simulink model "EcoSIM3_P2_C2"  (R2014b)
settings: Solver=ode1  SolverMode=SingleTasking  StartTime=0.0  StopTime=inf  FixedStep=0.01  RelTol=1e-3
PostLoadFcn:
  | %, if any(exist('dsrtsu_mdlpostloadfcn', 'file') == [2, 3, 6]), try dsrtsu_mdlpostloadfcn('Execute', bdroot); catch fprintf('Error in PostLoadFcn (dsrtsu_mdlpostloadfcn) for model "%s":\n %s\n', bdroot, lasterr); end, end,
InitFcn:
  | tic
  | %Startup_EcoSIM
values from neighbouring files (symbols this model uses):
  EngPwr = [0 5	10	15	20	25	30	35	40	45	50	55	60	65	70	75	80	85	90	95	100	105	110	115]    [Series_Maps.m]
  EngSpd = [0 477.4645 954.929 1909.858 2864.787 3819.716 4774.645 5729.574 6684.503]    [Series_Maps.m]
  EngTrq = [0	0	0	0	0	0	0	0	0	0	0	0	0	0	0	0	0	0	0	0	0	0	0	0 ... (first row only)    [Series_Maps.m]
  Power = [0 5 10 15 20 25 30]    [Series_Maps.m]
  Torque = [-50,-40,-30,-25,-20,-15,-10,-8,-6,-4,-2,0]    [Series_Maps.m]
undefined symbols (not defined in the file or in its folder): canChannel, Controls, DriveCycles, Driver, EM_EFF_MAP, EM_PwrLoss_MAP, Glbl, Plants, Veh_Dynamics
libraries: canmsglib x100, canlib x87, fl_lib x78, simulink x59, nesl_utility x40, sdl_lib x17, dspsigops x5, dspswit3 x3, dspstat3 x2, commnoisgen2 x1, dspfdesign x1
(part 5 of 15)

== system EcoSIM3_P2_C2/Powertrain/Electrical Storage System/Soft ECU/Outputs ==
  note: Select the Sensor signals
  From Algorithm : Inport
  Bus Creator2 : BusCreator  Inputs=6
  Bus Creator3 : BusCreator  Inputs=2
  Bus Selector : BusSelector  OutputSignals=AccPwrMdlHiVltInpCrnt,bcm_mainc_stat,Batt_SOC_percent,SoftECU_Out,Batt_Voltage_V,Batt_Current_A,bcm_cell_tmax,bcm_cell_tmin
  Actuator_Cmds : Outport
  To ECUs : Outport  Port=2
  wires:
  Bus Selector/4 -> Bus Creator2/2  "<SoftECU_Out>"
  Bus Selector/3 -> Bus Creator2/1  "<Batt_SOC_percent>"
  Bus Selector/2 -> Bus Creator3/2  "<bcm_mainc_stat>"
  Bus Selector/1 -> Bus Creator3/1  "<AccPwrMdlHiVltInpCrnt>"
  From Algorithm/1 -> Bus Selector/1
  Bus Creator2/1 -> To ECUs/1  "ESS_CAN_Out"
  Bus Creator3/1 -> Actuator_Cmds/1  "ESS_Actuator_Cmds"
  Bus Selector/5 -> Bus Creator2/3  "<Batt_Voltage_V>"
  Bus Selector/6 -> Bus Creator2/4  "<Batt_Current_A>"
  Bus Selector/7 -> Bus Creator2/5  "<bcm_cell_tmax>"
  Bus Selector/8 -> Bus Creator2/6  "<bcm_cell_tmin>"

== system EcoSIM3_P2_C2/Powertrain/Engine/ Component Model/Actuators ==
  note: Actuator Model or a Signal Pass-through, Remove the bus if you are passing through all the signals
  ActuatorInputs : Inport
  Actuator Outputs : Outport
  wires:
  ActuatorInputs/1 -> Actuator Outputs/1

== system EcoSIM3_P2_C2/Powertrain/Engine/ Component Model/Plant ==
  note: Component Level Performance Maps
  note: Three kinds of Outputs:
      | 1.To_sensors: Signals that can actually be sensed through Sensors go to sensor models
      | 2. To_plants: Signals that are not actually sensed by sensors but are utilized by the rest of the plant and actually happen physically
      | Component_Logging: Logs both the signal kinds before going through sensor
  From_Actuators : Inport
  Sensors_Feedback : Inport  Port=2
  Bus Selector : BusSelector  OutputSignals=ICE_Torque_Cmd_Nm
  Bus Selector1 : BusSelector  OutputSignals=ICE_Speed_rad_per_s
  Compare To Constant : simulink/Logic and Bit Operations/Compare To Constant  relop=>=  const=0  OutDataTypeStr=boolean
  Generic Engine : sdl_lib/Engines/Generic Engine  Commented=on  model_parameterization=1  engine_type=1  P_max=max(Plants.ICE.Mdl.Plant.Max_Trq.Trq.*Plants.ICE.Mdl.Plant.Max_Trq.w) W  w_P_max=6000 rpm  w_max="max(Plants.ICE.Mdl.Plant.Max_Trq.RPM)  rpm"  w_min="min(Plants.ICE.Mdl.Plant.Max_Trq.RPM)  rpm"  w_tab=[ 500 1000 2e+3 3e+3 4e+3 5e+3 6e+3 7e+3 ] rpm  trq_tab=[ 380 380 380 380 350 280 200 80 ] N*m  pwr_tab=[ 2e+4 4e+4 7.8e+4 1.2e+5 1.45e+5 1.48e+5 1.25e+5 6e+4 ] W  interp_method=1  model_inertia=0  inertia=1 kg*m^2  initial_velocity=800 rpm  model_time_constant=0  time_constant=0.2 s  T0=0  w_thr="max(Plants.ICE.Mdl.Plant.Max_Trq.RPM)  rpm"  idle_speed=1  idle_speed_reference="min(Plants.ICE.Mdl.Plant.Max_Trq.RPM)  rpm"  tau_controller=1 s  idle_w_thr=1 rpm  fc_model=2  fc_per_rev=25 mg/rev  displaced_volume=400 cm^3  rev_per_cycle=2  fc_w_tab=Plants.ICE.Mdl.Plant.m_dot.RPM rpm  fc_trq_tab=Plants.ICE.Mdl.Plant.m_dot.Trq N*m  fc_tab=Plants.ICE.Mdl.Plant.m_dot.fuel_kg_per_s'.*1000 g/s  bmep_tab=[ 0 250 500 625 750 1000 1.15e+3 1.25e+3 ] kPa  bsfc_tab=[ 410 380 300 280 270 290 320 380; 410 370 290 270 260 270 285 320; 415 380 290 275 265 270 270 300; 420 390 310 290 285 280 280 285; 430 410 340 320 310 300 310 320; 450 430 370 340 330 330 350 380 ] g/hr/kW  fc_interp_method=1
      settings: LogSimulationData=on
  ICE Friction Curve : Lookup  InputValues=Plants.ICE.Mdl.Plant.Friction_Trq.w  Table=Plants.ICE.Mdl.Plant.Friction_Trq.Trq  LookUpMeth=Interpolation-Use End Values  SaturateOnIntegerOverflow=on
  ICE Fuel Mass Flow Rate Map (kg/s) : Lookup2D  RowIndex=Plants.ICE.Mdl.Plant.m_dot.w  ColumnIndex=Plants.ICE.Mdl.Plant.m_dot.Trq  Table=Plants.ICE.Mdl.Plant.m_dot.fuel_kg_per_s'  LookUpMeth=Interpolation-Use End Values  SaturateOnIntegerOverflow=on  InputSameDT=on
  Ideal Torque Source : fl_lib/Mechanical/Mechanical Sources/Ideal Torque Source
  Ideal Torque Source1 : fl_lib/Mechanical/Mechanical Sources/Ideal Torque Source
  Inertia : fl_lib/Mechanical/Rotational Elements/Inertia  inertia=0.227 kg*m^2  w_specify=off  w_priority=High  w=0 rad/s  t_specify=off  t_priority=High  t=0 N*m
  Product : Product
  Reference : fl_lib/Mechanical/Rotational Elements/Mechanical Rotational Reference
  Reference1 : fl_lib/Mechanical/Rotational Elements/Mechanical Rotational Reference
  Simulink-PS Converter : nesl_utility/Simulink-PS Converter  PhysicalDomain=network_engine_domain  SubClassName=ps_input  LeftPortType=input  RightPortType=output  PseudoPeriodic=off  Frequencies=[]  NoiseDistribution=none  NoiseParameters=[]  Unit=N*m  AffineConversion=off  InputFiltering=off  SimscapeFilterOrder=1  InputFilterTimeConstant=0.001  UdotUserProvided=1
  Simulink-PS Converter1 : nesl_utility/Simulink-PS Converter  PhysicalDomain=network_engine_domain  SubClassName=ps_input  LeftPortType=input  RightPortType=output  PseudoPeriodic=off  Frequencies=[]  NoiseDistribution=none  NoiseParameters=[]  Unit=N*m  AffineConversion=off  InputFiltering=off  SimscapeFilterOrder=1  InputFilterTimeConstant=0.001  UdotUserProvided=1
  ICE Output Shaft : PMIOPort  Tag=PMCPort  Port=1  Side=Right
  Fuel_Consumtion_kg_per_s : Outport
  wires:
  From_Actuators/1 -> Bus Selector/1
  ICE Fuel Mass Flow Rate Map (kg/s)/1 -> Fuel_Consumtion_kg_per_s/1  "ICE_m_f_dot_kg_per_s"
  Bus Selector1/1 -> Compare To Constant/1, ICE Friction Curve/1, ICE Fuel Mass Flow Rate Map (kg/s)/1  "<ICE_Speed_rad_per_s>"
  Sensors_Feedback/1 -> Bus Selector1/1
  ICE Friction Curve/1 -> Product/2
  Bus Selector/1 -> Simulink-PS Converter/1, ICE Fuel Mass Flow Rate Map (kg/s)/2  "<ICE_Torque_Cmd_Nm>"
  Compare To Constant/1 -> Product/1
  Product/1 -> Simulink-PS Converter1/1
  connections:
  Simulink-PS Converter/RConn1 -- Ideal Torque Source/RConn1
  Reference/LConn1 -- Ideal Torque Source/RConn2
  ICE Output Shaft/RConn1 -- Ideal Torque Source/LConn1 -- Inertia/LConn1 -- Ideal Torque Source1/LConn1
  Reference1/LConn1 -- Ideal Torque Source1/RConn2
  Simulink-PS Converter1/RConn1 -- Ideal Torque Source1/RConn1

== system EcoSIM3_P2_C2/Powertrain/Engine/ Component Model/Sensors ==
  note: Sensor Model: Place where we add Corrupter
  Fuel_Consumption : Inport
  Bus Creator : BusCreator  Inputs=3
  Gain : Gain  Gain=9.549
  Ideal Rotational Motion Sensor : fl_lib/Mechanical/Mechanical Sensors/Ideal Rotational Motion Sensor  offset=0 rad
  Ideal Torque Sensor : fl_lib/Mechanical/Mechanical Sensors/Ideal Torque Sensor
  Mechanical Rotational Reference1 : fl_lib/Mechanical/Rotational Elements/Mechanical Rotational Reference
  PS-Simulink Converter : nesl_utility/PS-Simulink Converter  PhysicalDomain=network_engine_domain  SubClassName=ps_output  LeftPortType=input  RightPortType=output  PseudoPeriodic=off  Frequencies=[]  Unit=1  AffineConversion=off
  PS-Simulink Converter1 : nesl_utility/PS-Simulink Converter  PhysicalDomain=network_engine_domain  SubClassName=ps_output  LeftPortType=input  RightPortType=output  PseudoPeriodic=off  Frequencies=[]  Unit=N*m  AffineConversion=off
  Product : Product
  Scope : Scope
      settings: YMin=480  YMax=600  SaveName=ScopeData16
  Sensor lag : Subsystem
  Sensor lag1 : Subsystem
  Terminator : Terminator
  ICE_Ouput_Shaft : PMIOPort  Port=1  Side=Left
  To_Belt : PMIOPort  Port=2  Side=Right
  Sensor Out : Outport
  Fuel : Outport  Port=2
  wires:
  Bus Creator/1 -> Sensor Out/1  "ICE_Sensor_Out"
  Sensor lag/1(o) -> Product/1, Bus Creator/1  "ICE_Speed_rad_per_s"
  Sensor lag1/1(o) -> Product/2, Bus Creator/2  "Engine_Torque_Out_Nm"
  Fuel_Consumption/1 -> Fuel/1, Bus Creator/3  "ICE_m_f_dot_kg_per_s"
  PS-Simulink Converter/1 -> Gain/1, Sensor lag/1(i)  "ICE_Speed_rad_per_s"
  PS-Simulink Converter1/1 -> Sensor lag1/1(i)  "Engine_Torque_Out_Nm"
  Product/1 -> Terminator/1
  Gain/1 -> Scope/1
  connections:
  ICE_Ouput_Shaft/RConn1 -- Ideal Torque Sensor/LConn1 -- Ideal Rotational Motion Sensor/LConn1
  Ideal Rotational Motion Sensor/RConn1 -- Mechanical Rotational Reference1/LConn1
  PS-Simulink Converter/LConn1 -- Ideal Rotational Motion Sensor/RConn2
  PS-Simulink Converter1/LConn1 -- Ideal Torque Sensor/RConn2
  To_Belt/RConn1 -- Ideal Torque Sensor/RConn1

== system EcoSIM3_P2_C2/Powertrain/Engine/Soft ECU/Algorithm ==
  note: Signals like T& E are used to calculate whatever is required by Soft ECU
  note: Sensor signals getting transmitted over CAN are selected here
  note: Sensor signals getting transmitted over CAN are bussed together here
  note: Signals getting transmitted to Actuators are bussed together here
  Inputs : Inport
  Bus Selector : BusSelector  OutputSignals=ICE_Sensor_Out,ECM_SoftECU_Receive.ICE_Electrical.ICE_Powerup,ECM_SoftECU_Receive.ICE_CAN.ICE_Request.ICE_Torque_Request_Nm,ECM_SoftECU_Receive.ICE_CAN.ICE_Request.PCM_Wake,ECM_SoftECU_Receive.ICE_CAN.ICE_Request.ISP_R,ICE_Sensor_Out.ICE_Speed_rad_per_s
  Bus Selector1 : BusSelector  OutputSignals=ICE_Speed_rad_per_s
  Constant : Constant  Value=Plants.ICE.Mdl.Plant.red_line_w
  ECM SoftECU : Stateflow chart  TreatAsAtomicUnit=on
  ICE Friction Curve : Lookup  InputValues=Plants.ICE.Mdl.Plant.Friction_Trq.w  Table=Plants.ICE.Mdl.Plant.Friction_Trq.Trq  LookUpMeth=Interpolation-Use End Values  SaturateOnIntegerOverflow=on
  ICE Max Torque Curve : Lookup  InputValues=Plants.ICE.Mdl.Plant.Max_Trq.w  Table=Plants.ICE.Mdl.Plant.Max_Trq.Trq  LookUpMeth=Interpolation-Use End Values  SaturateOnIntegerOverflow=on
  Saturation Dynamic : simulink/Discontinuities/Saturation Dynamic  OutMin=[]  OutMax=[]  OutDataTypeStr=Inherit: Same as second input  OutDataType=sfix(16)  OutScaling=2^-10  DoSatur=off
  Outputs : Outport  OutputWhenDisabled=reset  InitialOutput=0
  wires:
  Inputs/1 -> Bus Selector/1
  Bus Selector/1 -> Bus Selector1/1  "<ICE_Sensor_Out>"
  Bus Selector1/1 -> ICE Max Torque Curve/1, ECM SoftECU/1(Engine_Speed)  "<ICE_Speed_rad_per_s>"
  Bus Selector/3 -> ECM SoftECU/3(Torque_Request)  "<ICE_Torque_Request_Nm>"
  ICE Friction Curve/1 -> Saturation Dynamic/3
  ICE Max Torque Curve/1 -> Saturation Dynamic/1
  Saturation Dynamic/1 -> Outputs/1  "ICE_Torque_Cmd_Nm"
  ECM SoftECU/1(Torque_Cmd) -> Saturation Dynamic/2
  Bus Selector/2 -> ECM SoftECU/2(ECM_Powerup)  "<ICE_Powerup>"
  Bus Selector/4 -> ECM SoftECU/4(PCM_Wake)  "<PCM_Wake>"
  Bus Selector/5 -> ECM SoftECU/5(ISP_R)  "<ISP_R>"
  Bus Selector/6 -> ICE Friction Curve/1  "<ICE_Speed_rad_per_s>"
  Constant/1 -> ECM SoftECU/6(Max_Speed)

== system EcoSIM3_P2_C2/Powertrain/Engine/Soft ECU/Inputs ==
  note: Do the input conditioning (if any) required by the
      | Algorith
  note: Select the CAN signals
  note: Select the Sensor signals
  note: Combine all the Signals that go to the
      | Soft ECU Algorithm:
      | -Calculated Signals from Sensors and CAN
      | -Signalfrom sensors pass through because they
      | need to be sent out over the CAN by the ECU
  ICE_In : Inport
  Sensors : Inport  Port=2
  Bus Creator : BusCreator  Inputs=3
  Bus Selector : BusSelector  OutputSignals=ECM_SoftECU_Receive
  Bus Selector1 : BusSelector  OutputSignals=ICE_Speed_rad_per_s
  To_Algorithm : Outport
  wires:
  ICE_In/1 -> Bus Selector/1
  Sensors/1 -> Bus Creator/1, Bus Selector1/1  "ICE_Sensor_Out"
  Bus Creator/1 -> To_Algorithm/1  "Component_to_Alg"
  Bus Selector/1 -> Bus Creator/3  "<ECM_SoftECU_Receive>"
  Bus Selector1/1 -> Bus Creator/2  "<ICE_Speed_rad_per_s>"

== system EcoSIM3_P2_C2/Powertrain/Engine/Soft ECU/Inputs1 ==
  note: Combine all the Signals that go to the
      | Soft ECU Algorithm:
      | -Calculated Signals from Sensors and CAN
      | -Signalfrom sensors pass through because they
      | need to be sent out over the CAN by the ECU
  note: Select the CAN signals
  note: Do the input conditioning (if any) required by the
      | Algorith
  From Algorithm : Inport
  Bus Creator : BusCreator  Inputs=1
  Bus Creator1 : BusCreator  Inputs=1
  ICE_Out : Outport
  Actuator Cmds : Outport  Port=2
  wires:
  Bus Creator/1 -> ICE_Out/1  "ICE_CAN_Out"
  Bus Creator1/1 -> Actuator Cmds/1  "ICE_Actuator_Cmds"
  From Algorithm/1 -> Bus Creator/1, Bus Creator1/1

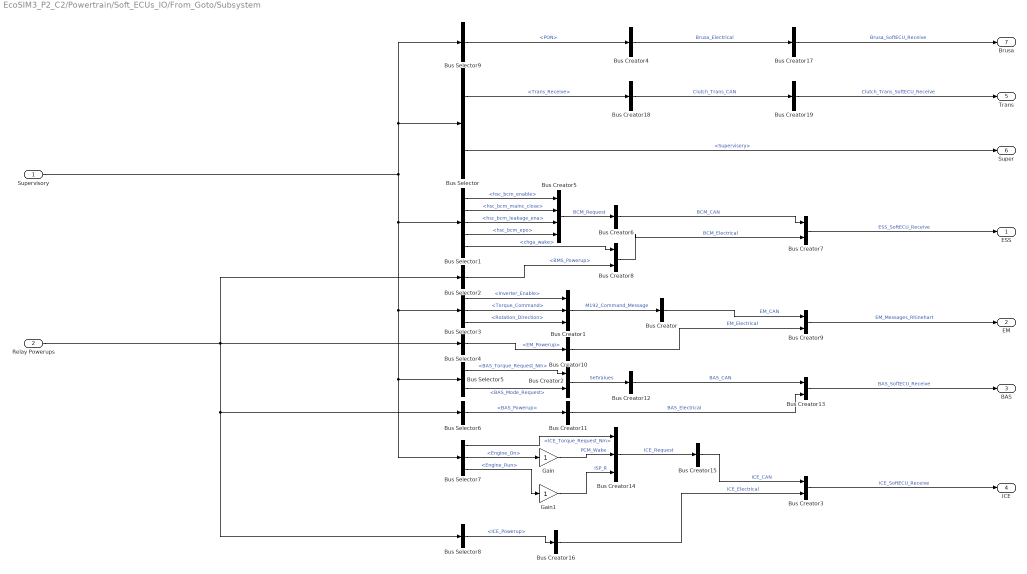
== system EcoSIM3_P2_C2/Powertrain/Soft_ECUs_IO/From_Goto/Subsystem ==
  Supervisory : Inport
  Relay Powerups : Inport  Port=2
  Bus Creator{,4,6,10..12,15..19} (11 alike) : BusCreator  Inputs=1
  Bus Creator1 : BusCreator  Inputs=3
  Bus Creator{2..3,7..9,13} (6 alike) : BusCreator  Inputs=2
  Bus Creator14 : BusCreator  Inputs=3
  Bus Creator5 : BusCreator
  Bus Selector : BusSelector  OutputSignals=Supervisory_Requests.Supervisory_CAN.Trans_Receive,Supervisory_Requests.Supervisory_CAN.Supervisory
  Bus Selector1 : BusSelector  OutputSignals=Supervisory_Requests.Supervisory_CAN.ESS_Signals_A123.hsc_bcm_enable,Supervisory_Requests.Supervisory_CAN.ESS_Signals_A123.hsc_bcm_mainc_close,Supervisory_Requests.Supervisory_CAN.ESS_Signals_A123.hsc_bcm_leakage_ena,Supervisory_Requests.Supervisory_CAN.ESS_Signals_A123.hsc_bcm_epo,Supervisory_Requests.Supervisory_Electrical.chga_wake
  Bus Selector2 : BusSelector  OutputSignals=BMS_Powerup
  Bus Selector3 : BusSelector  OutputSignals=Supervisory_Requests.Supervisory_CAN.EM_Messages_Rhinehart.Inverter_Enable,Supervisory_Requests.Supervisory_CAN.EM_Messages_Rhinehart.Torque_Command,Supervisory_Requests.Supervisory_CAN.EM_Messages_Rhinehart.Rotation_Direction
  Bus Selector4 : BusSelector  OutputSignals=EM_Powerup
  Bus Selector5 : BusSelector  OutputSignals=Supervisory_Requests.Supervisory_CAN.BAS_SoftECU_Receive.BAS_Torque_Request_Nm,Supervisory_Requests.Supervisory_CAN.BAS_SoftECU_Receive.BAS_Mode_Request
  Bus Selector6 : BusSelector  OutputSignals=BAS_Powerup
  Bus Selector7 : BusSelector  OutputSignals=Supervisory_Requests.Supervisory_CAN.Engine_Messages.ICE_Torque_Request_Nm,Supervisory_Requests.Supervisory_CAN.Engine_Messages.Engine_On,Supervisory_Requests.Supervisory_CAN.Engine_Messages.Engine_Run
  Bus Selector8 : BusSelector  OutputSignals=ICE_Powerup
  Bus Selector9 : BusSelector  OutputSignals=Supervisory_Requests.Supervisory_Electrical.PON
  Gain : Gain
  Gain1 : Gain
  ESS : Outport
  EM : Outport  Port=2  SampleTime=0.01
  BAS : Outport  Port=3
  ICE : Outport  Port=4
  Trans : Outport  Port=5
  Super : Outport  Port=6
  Brusa : Outport  Port=7
  wires:
  Bus Selector/2 -> Super/1  "<Supervisory>"
  Bus Selector/1 -> Bus Creator18/1  "<Trans_Receive>"
  Supervisory/1 -> Bus Selector7/1, Bus Selector5/1, Bus Selector3/1, Bus Selector1/1, Bus Selector9/1, Bus Selector/1
  Bus Selector1/3 -> Bus Creator5/3  "<hsc_bcm_leakage_ena>"
  Bus Selector1/1 -> Bus Creator5/1  "<hsc_bcm_enable>"
  Bus Selector1/2 -> Bus Creator5/2  "<hsc_bcm_mainc_close>"
  Bus Selector1/4 -> Bus Creator5/4  "<hsc_bcm_epo>"
  Relay Powerups/1 -> Bus Selector2/1, Bus Selector8/1, Bus Selector6/1, Bus Selector4/1
  Bus Selector2/1 -> Bus Creator8/2  "<BMS_Powerup>"
  Bus Selector3/3 -> Bus Creator1/3  "<Rotation_Direction>"
  Bus Selector3/1 -> Bus Creator1/1  "<Inverter_Enable>"
  Bus Selector3/2 -> Bus Creator1/2  "<Torque_Command>"
  Bus Selector4/1 -> Bus Creator10/1  "<EM_Powerup>"
  Bus Selector5/1 -> Bus Creator2/1  "<BAS_Torque_Request_Nm>"
  Bus Selector5/2 -> Bus Creator2/2  "<BAS_Mode_Request>"
  Bus Selector6/1 -> Bus Creator11/1  "<BAS_Powerup>"
  Bus Creator9/1 -> EM/1  "EM_Messages_Rhinehart"
  Bus Creator13/1 -> BAS/1  "BAS_SoftECU_Receive"
  Bus Creator3/1 -> ICE/1  "ICE_SoftECU_Receive"
  Bus Selector7/1 -> Bus Creator14/1  "<ICE_Torque_Request_Nm>"
  Bus Selector8/1 -> Bus Creator16/1  "<ICE_Powerup>"
  Bus Selector1/5 -> Bus Creator8/1  "<chga_wake>"
  Bus Selector9/1 -> Bus Creator4/1  "<PON>"
  Bus Creator4/1 -> Bus Creator17/1  "Brusa_Electrical"
  Bus Creator5/1 -> Bus Creator6/1  "BCM_Request"
  Bus Creator6/1 -> Bus Creator7/1  "BCM_CAN"
  Bus Creator8/1 -> Bus Creator7/2  "BCM_Electrical"
  Bus Creator7/1 -> ESS/1  "ESS_SoftECU_Receive"
  Bus Creator1/1 -> Bus Creator/1  "M192_Command_Message"
  Bus Creator/1 -> Bus Creator9/1  "EM_CAN"
  Bus Creator10/1 -> Bus Creator9/2  "EM_Electrical"
  Bus Creator2/1 -> Bus Creator12/1  "SetValues"
  Bus Creator12/1 -> Bus Creator13/1  "BAS_CAN"
  Bus Creator11/1 -> Bus Creator13/2  "BAS_Electrical"
  Bus Creator14/1 -> Bus Creator15/1  "ICE_Request"
  Bus Creator15/1 -> Bus Creator3/1  "ICE_CAN"
  Bus Creator16/1 -> Bus Creator3/2  "ICE_Electrical"
  Bus Creator17/1 -> Brusa/1  "Brusa_SoftECU_Receive"
  Bus Creator18/1 -> Bus Creator19/1  "Clutch_Trans_CAN"
  Bus Creator19/1 -> Trans/1  "Clutch_Trans_SoftECU_Receive"
  Bus Selector7/3 -> Gain1/1  "<Engine_Run>"
  Bus Selector7/2 -> Gain/1  "<Engine_On>"
  Gain/1 -> Bus Creator14/2  "PCM_Wake"
  Gain1/1 -> Bus Creator14/3  "ISP_R"

== system EcoSIM3_P2_C2/Powertrain/Soft_ECUs_IO/From_Goto/Subsystem1 ==
  note: Components with Relay:
      | On Charging Relay:
      | MABx
      | A123
      | DC-DC
      |
      | On Vehicle Relay:
      | MABx
      | A123
      | DC-DC
      | EM
      | BAS
      | Engine
      | Accessories other than DC-DC (for this model HVAC)
  From_GCM : Inport
  BAS_Relay : Subsystem
  Bus Creator1 : BusCreator
  Bus Selector : BusSelector  OutputSignals=GCM_Electrical_Out.Relay_Charge,GCM_Electrical_Out.Relay_Vehicle
  Constant : Constant
  Constant1 : Constant  Value=0
  Constant10 : Constant  Value=0
  Constant9 : Constant
  EM_Relay : Subsystem
  Engine_Relay : Subsystem
  Relay : Switch  Criteria=u2 > Threshold  Threshold=0.5
  Relay4 : Switch  Criteria=u2 > Threshold  Threshold=0.5
  SoftECUPowerup : Outport
  MABxPowerup : Outport  Port=2
  wires:
  Constant9/1 -> Relay4/1
  Bus Selector/2 -> BAS_Relay/1(In1), Engine_Relay/1(In1), EM_Relay/1(In1)  "<Relay_Vehicle>"
  Relay4/1 -> MABxPowerup/1  "Supervisory_Wakeup"
  Constant/1 -> Relay/1
  Bus Creator1/1 -> SoftECUPowerup/1  "Powerups"
  Constant10/1 -> Relay4/3
  Bus Selector/1 -> Relay4/2, Relay/2  "<Relay_Charge>"
  Constant1/1 -> Relay/3
  From_GCM/1 -> Bus Selector/1
  BAS_Relay/1(Out1) -> Bus Creator1/4
  Engine_Relay/1(Out1) -> Bus Creator1/3
  EM_Relay/1(Out1) -> Bus Creator1/2
  Relay/1 -> Bus Creator1/1  "BMS_Powerup"

== system EcoSIM3_P2_C2/Powertrain/Soft_ECUs_IO/VNT Kvaser/CANRx ==
  BAS Receive : Subsystem
  Brusa Receive : Subsystem
  Bus Creator : BusCreator  Inputs=7
  EM Receive : Subsystem
  ESS Receive : Subsystem
  ICE Receive : Subsystem
  Transmisssion Receive : Subsystem
  CAN Out : Outport
  wires:
  Bus Creator/1 -> CAN Out/1  "CANRx"
  ESS Receive/1(ESS CAN) -> Bus Creator/4
  Transmisssion Receive/2(Mode) -> Bus Creator/3
  Transmisssion Receive/1(Clutch_Trans) -> Bus Creator/2
  ICE Receive/1(ICE CAN) -> Bus Creator/7
  BAS Receive/1(BAS_CAN) -> Bus Creator/6
  EM Receive/1(EM CAN) -> Bus Creator/5
  Brusa Receive/1(Brusa CAN) -> Bus Creator/1

== system EcoSIM3_P2_C2/Powertrain/Soft_ECUs_IO/VNT Kvaser/CANTx ==
  CAN : Inport
  BAS : Subsystem
  Brusa : Subsystem
  Bus Selector : BusSelector  OutputSignals=ESS_CAN_Out,EM_CAN_Out,ICE_CAN_Out,Clutch_Transmission_CAN_Out,GMLAN_CAN_Out,BAS_CAN_Out,Brusa_CAN_Out
  Clutch_and_Trans : Subsystem
  EM : Subsystem
  ESS : Subsystem
  Engine : Subsystem
  GMLAN : Subsystem
  wires:
  Bus Selector/6 -> BAS/1(BAS)  "<BAS_CAN_Out>"
  Bus Selector/5 -> GMLAN/1(Driver)  "<GMLAN_CAN_Out>"
  Bus Selector/4 -> Clutch_and_Trans/1(Trans)  "<Clutch_Transmission_CAN_Out>"
  Bus Selector/3 -> Engine/1(ICE)  "<ICE_CAN_Out>"
  Bus Selector/2 -> EM/1(EM)  "<EM_CAN_Out>"
  Bus Selector/1 -> ESS/1(ESS)  "<ESS_CAN_Out>"
  CAN/1 -> Bus Selector/1
  Bus Selector/7 -> Brusa/1(Brusa)  "<Brusa_CAN_Out>"

== system EcoSIM3_P2_C2/Powertrain/Soft_ECUs_IO/VNT Kvaser/ElectricalRx ==
  note: Components with Relay:
      | On Charging Relay:
      | MABx
      | A123
      | DC-DC
      |
      | On Vehicle Relay:
      | MABx
      | A123
      | DC-DC
      | EM
      | BAS
      | Engine
      | Accessories other than DC-DC (for this model HVAC)
  BAS_Relay : Subsystem
  Bus Creator : BusCreator  Inputs=2
  Bus Creator1 : BusCreator  Inputs=6
  Bus Creator{2,4,10..11,16} (5 alike) : BusCreator  Inputs=1
  Bus Creator8 : BusCreator  Inputs=2
  Bus Selector : BusSelector  OutputSignals=Supervisory_Electrical_Out.PON,Supervisory_Electrical_Out.chga_wake,GCM_Electrical_Out.Relay_Charge,GCM_Electrical_Out.Relay_Vehicle
  Constant : Constant
  Constant1 : Constant  Value=0
  Constant10 : Constant  Value=0
  Constant9 : Constant
  EM_Relay : Subsystem
  Engine_Relay : Subsystem
  Ground : Ground
  Relay : Switch  Criteria=u2 > Threshold  Threshold=0.5
  Relay4 : Switch  Criteria=u2 > Threshold  Threshold=0.5
  Terminator : Terminator
  Electrical : Outport
  wires:
  [VNT_Electrical_FromMABx] -> Bus Creator/1
  [VNT_Electrical_FromGCM] -> Bus Creator/2
  Bus Selector/2 -> Bus Creator8/1  "<chga_wake>"
  Relay/1 -> Bus Creator8/2  "BMS_Powerup"
  Bus Creator8/1 -> Bus Creator1/3  "BCM_Electrical"
  Constant9/1 -> Relay4/1
  Bus Selector/4 -> EM_Relay/1(In1), Engine_Relay/1(In1), BAS_Relay/1(In1)  "<Relay_Vehicle>"
  Relay4/1 -> Terminator/1  "Supervisory_Wakeup"
  Constant/1 -> Relay/1
  Constant10/1 -> Relay4/3
  Bus Selector/3 -> Relay/2, Relay4/2  "<Relay_Charge>"
  Constant1/1 -> Relay/3
  Bus Creator/1 -> Bus Selector/1
  Bus Selector/1 -> Bus Creator4/1  "<PON>"
  Bus Creator4/1 -> Bus Creator1/2  "Brusa_Electrical"
  Bus Creator2/1 -> Bus Creator1/1  "Clutch_Trans_Electrical"
  Ground/1 -> Bus Creator2/1  "Dummy1"
  EM_Relay/1(Out1) -> Bus Creator10/1
  Bus Creator10/1 -> Bus Creator1/4  "EM_Electrical"
  Bus Creator11/1 -> Bus Creator1/6  "BAS_Electrical"
  BAS_Relay/1(Out1) -> Bus Creator11/1
  Bus Creator16/1 -> Bus Creator1/5  "ICE_Electrical"
  Engine_Relay/1(Out1) -> Bus Creator16/1
  Bus Creator1/1 -> Electrical/1  "ElectricalRx"

== system EcoSIM3_P2_C2/Powertrain/Soft_ECUs_IO/VNT Kvaser/ElectricalTx ==
  Electrical : Inport
  Bus Creator : BusCreator  Inputs=7
  Bus Selector1 : BusSelector  OutputSignals=Brusa_Electrical_Out,Clutch_Transmission_Electrical_Out,GM_Electrical_Out,ESS_Electrical_Out,EM_Electrical_Out,BAS_Electrical_Out,ICE_Electrical_Out
  tag scope: VNT_Electrical_From_SoftECU=global
  wires:
  Electrical/1 -> Bus Selector1/1
  Bus Selector1/5 -> Bus Creator/5  "<EM_Electrical_Out>"
  Bus Selector1/6 -> Bus Creator/6  "<BAS_Electrical_Out>"
  Bus Selector1/3 -> Bus Creator/3  "<GM_Electrical_Out>"
  Bus Selector1/7 -> Bus Creator/7  "<ICE_Electrical_Out>"
  Bus Selector1/4 -> Bus Creator/4  "<ESS_Electrical_Out>"
  Bus Selector1/1 -> Bus Creator/1  "<Brusa_Electrical_Out>"
  Bus Selector1/2 -> Bus Creator/2  "<Clutch_Transmission_Electrical_Out>"
  Bus Creator/1 -> [VNT_Electrical_From_SoftECU]  "From_SoftECU"

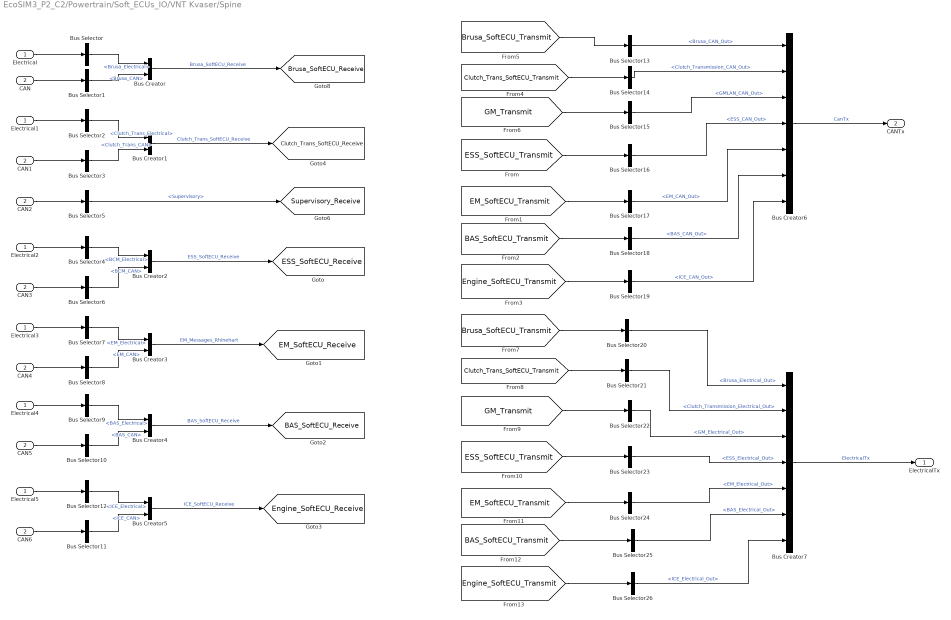
== system EcoSIM3_P2_C2/Powertrain/Soft_ECUs_IO/VNT Kvaser/Spine ==
  Electrical : Inport
  CAN : Inport  Port=2
  Bus Creator{,1..5} (6 alike) : BusCreator  Inputs=2
  Bus Creator6 : BusCreator  Inputs=7
  Bus Creator7 : BusCreator  Inputs=7
  Bus Selector : BusSelector  OutputSignals=Brusa_Electrical
  Bus Selector1 : BusSelector  OutputSignals=Brusa_CAN
  Bus Selector10 : BusSelector  OutputSignals=BAS_CAN
  Bus Selector11 : BusSelector  OutputSignals=ICE_CAN
  Bus Selector12 : BusSelector  OutputSignals=ICE_Electrical
  Bus Selector13 : BusSelector  OutputSignals=Brusa_CAN_Out
  Bus Selector14 : BusSelector  OutputSignals=Clutch_Transmission_CAN_Out
  Bus Selector15 : BusSelector  OutputSignals=GMLAN_CAN_Out
  Bus Selector16 : BusSelector  OutputSignals=ESS_CAN_Out
  Bus Selector17 : BusSelector  OutputSignals=EM_CAN_Out
  Bus Selector18 : BusSelector  OutputSignals=BAS_CAN_Out
  Bus Selector19 : BusSelector  OutputSignals=ICE_CAN_Out
  Bus Selector2 : BusSelector  OutputSignals=Clutch_Trans_Electrical
  Bus Selector20 : BusSelector  OutputSignals=Brusa_Electrical_Out
  Bus Selector21 : BusSelector  OutputSignals=Clutch_Transmission_Electrical_Out
  Bus Selector22 : BusSelector  OutputSignals=GM_Electrical_Out
  Bus Selector23 : BusSelector  OutputSignals=ESS_Electrical_Out
  Bus Selector24 : BusSelector  OutputSignals=EM_Electrical_Out
  Bus Selector25 : BusSelector  OutputSignals=BAS_Electrical_Out
  Bus Selector26 : BusSelector  OutputSignals=ICE_Electrical_Out
  Bus Selector3 : BusSelector  OutputSignals=Clutch_Trans_CAN
  Bus Selector4 : BusSelector  OutputSignals=BCM_Electrical
  Bus Selector5 : BusSelector  OutputSignals=Supervisory
  Bus Selector6 : BusSelector  OutputSignals=BCM_CAN
  Bus Selector7 : BusSelector  OutputSignals=EM_Electrical
  Bus Selector8 : BusSelector  OutputSignals=EM_CAN
  Bus Selector9 : BusSelector  OutputSignals=BAS_Electrical
  CAN{1..6} (6 alike) : InportShadow  Port=2
  Electrical{1..5} (5 alike) : InportShadow
  ElectricalTx : Outport
  CANTx : Outport  Port=2
  tag scope: BAS_SoftECU_Receive=global, Brusa_SoftECU_Receive=global, Clutch_Trans_SoftECU_Receive=global, EM_SoftECU_Receive=global, ESS_SoftECU_Receive=global, Engine_SoftECU_Receive=global, Supervisory_Receive=global
  wires:
  Electrical/1 -> Bus Selector/1
  CAN/1 -> Bus Selector1/1
  Bus Selector/1 -> Bus Creator/1  "<Brusa_Electrical>"
  Bus Selector1/1 -> Bus Creator/2  "<Brusa_CAN>"
  Bus Creator/1 -> [Brusa_SoftECU_Receive]  "Brusa_SoftECU_Receive"
  Electrical1/1 -> Bus Selector2/1
  CAN1/1 -> Bus Selector3/1
  Bus Selector2/1 -> Bus Creator1/1  "<Clutch_Trans_Electrical>"
  Bus Selector3/1 -> Bus Creator1/2  "<Clutch_Trans_CAN>"
  Bus Creator1/1 -> [Clutch_Trans_SoftECU_Receive]  "Clutch_Trans_SoftECU_Receive"
  CAN2/1 -> Bus Selector5/1
  Bus Selector5/1 -> [Supervisory_Receive]  "<Supervisory>"
  Electrical2/1 -> Bus Selector4/1
  CAN3/1 -> Bus Selector6/1
  Bus Selector4/1 -> Bus Creator2/1  "<BCM_Electrical>"
  Bus Selector6/1 -> Bus Creator2/2  "<BCM_CAN>"
  Bus Creator2/1 -> [ESS_SoftECU_Receive]  "ESS_SoftECU_Receive"
  Electrical3/1 -> Bus Selector7/1
  CAN4/1 -> Bus Selector8/1
  Bus Selector7/1 -> Bus Creator3/1  "<EM_Electrical>"
  Bus Selector8/1 -> Bus Creator3/2  "<EM_CAN>"
  Bus Creator3/1 -> [EM_SoftECU_Receive]  "EM_Messages_Rhinehart"
  Electrical4/1 -> Bus Selector9/1
  CAN5/1 -> Bus Selector10/1
  Bus Selector9/1 -> Bus Creator4/1  "<BAS_Electrical>"
  Bus Selector10/1 -> Bus Creator4/2  "<BAS_CAN>"
  Bus Creator4/1 -> [BAS_SoftECU_Receive]  "BAS_SoftECU_Receive"
  Electrical5/1 -> Bus Selector12/1
  CAN6/1 -> Bus Selector11/1
  Bus Selector12/1 -> Bus Creator5/1  "<ICE_Electrical>"
  Bus Selector11/1 -> Bus Creator5/2  "<ICE_CAN>"
  Bus Creator5/1 -> [Engine_SoftECU_Receive]  "ICE_SoftECU_Receive"
  [Brusa_SoftECU_Transmit] -> Bus Selector13/1
  [Clutch_Trans_SoftECU_Transmit] -> Bus Selector14/1
  [GM_Transmit] -> Bus Selector15/1
  [ESS_SoftECU_Transmit] -> Bus Selector16/1
  [EM_SoftECU_Transmit] -> Bus Selector17/1
  [BAS_SoftECU_Transmit] -> Bus Selector18/1
  [Engine_SoftECU_Transmit] -> Bus Selector19/1
  Bus Selector13/1 -> Bus Creator6/1  "<Brusa_CAN_Out>"
  Bus Selector14/1 -> Bus Creator6/2  "<Clutch_Transmission_CAN_Out>"
  Bus Selector15/1 -> Bus Creator6/3  "<GMLAN_CAN_Out>"
  Bus Selector16/1 -> Bus Creator6/4  "<ESS_CAN_Out>"
  Bus Selector17/1 -> Bus Creator6/5  "<EM_CAN_Out>"
  Bus Selector18/1 -> Bus Creator6/6  "<BAS_CAN_Out>"
  Bus Selector19/1 -> Bus Creator6/7  "<ICE_CAN_Out>"
  [Brusa_SoftECU_Transmit] -> Bus Selector20/1
  [Clutch_Trans_SoftECU_Transmit] -> Bus Selector21/1
  [GM_Transmit] -> Bus Selector22/1
  [ESS_SoftECU_Transmit] -> Bus Selector23/1
  [EM_SoftECU_Transmit] -> Bus Selector24/1
  [BAS_SoftECU_Transmit] -> Bus Selector25/1
  [Engine_SoftECU_Transmit] -> Bus Selector26/1
  Bus Selector20/1 -> Bus Creator7/1  "<Brusa_Electrical_Out>"
  Bus Selector21/1 -> Bus Creator7/2  "<Clutch_Transmission_Electrical_Out>"
  Bus Selector22/1 -> Bus Creator7/3  "<GM_Electrical_Out>"
  Bus Selector23/1 -> Bus Creator7/4  "<ESS_Electrical_Out>"
  Bus Selector24/1 -> Bus Creator7/5  "<EM_Electrical_Out>"
  Bus Selector25/1 -> Bus Creator7/6  "<BAS_Electrical_Out>"
  Bus Selector26/1 -> Bus Creator7/7  "<ICE_Electrical_Out>"
  Bus Creator7/1 -> ElectricalTx/1  "ElectricalTx"
  Bus Creator6/1 -> CANTx/1  "CanTx"

== system EcoSIM3_P2_C2/Powertrain/Soft_ECUs_IO/VNT Vector/CANRx ==
  BAS Receive : Subsystem
  Brusa Receive : Subsystem
  Bus Creator : BusCreator  Inputs=7
  EM Receive : Subsystem
  ESS Receive : Subsystem
  ICE Receive : Subsystem
  Transmisssion Receive : Subsystem
  CAN Out : Outport
  wires:
  Bus Creator/1 -> CAN Out/1  "CANRx"
  ESS Receive/1(ESS CAN) -> Bus Creator/4
  Transmisssion Receive/2(Mode) -> Bus Creator/3
  Transmisssion Receive/1(Clutch_Trans) -> Bus Creator/2
  ICE Receive/1(ICE CAN) -> Bus Creator/7
  BAS Receive/1(BAS_CAN) -> Bus Creator/6
  EM Receive/1(EM CAN) -> Bus Creator/5
  Brusa Receive/1(Brusa CAN) -> Bus Creator/1

== system EcoSIM3_P2_C2/Powertrain/Soft_ECUs_IO/VNT Vector/CANTx ==
  CAN : Inport
  BAS : Subsystem
  Brusa : Subsystem
  Bus Selector : BusSelector  OutputSignals=ESS_CAN_Out,EM_CAN_Out,ICE_CAN_Out,Clutch_Transmission_CAN_Out,GMLAN_CAN_Out,BAS_CAN_Out,Brusa_CAN_Out
  Clutch_and_Trans : Subsystem
  EM : Subsystem
  ESS : Subsystem
  Engine : Subsystem
  GMLAN : Subsystem
  wires:
  Bus Selector/6 -> BAS/1(BAS)  "<BAS_CAN_Out>"
  Bus Selector/5 -> GMLAN/1(Driver)  "<GMLAN_CAN_Out>"
  Bus Selector/4 -> Clutch_and_Trans/1(Trans)  "<Clutch_Transmission_CAN_Out>"
  Bus Selector/3 -> Engine/1(ICE)  "<ICE_CAN_Out>"
  Bus Selector/2 -> EM/1(EM)  "<EM_CAN_Out>"
  Bus Selector/1 -> ESS/1(ESS)  "<ESS_CAN_Out>"
  CAN/1 -> Bus Selector/1
  Bus Selector/7 -> Brusa/1(Brusa)  "<Brusa_CAN_Out>"

== system EcoSIM3_P2_C2/Powertrain/Soft_ECUs_IO/VNT Vector/ElectricalRx ==
  note: Components with Relay:
      | On Charging Relay:
      | MABx
      | A123
      | DC-DC
      |
      | On Vehicle Relay:
      | MABx
      | A123
      | DC-DC
      | EM
      | BAS
      | Engine
      | Accessories other than DC-DC (for this model HVAC)
  BAS_Relay : Subsystem
  Bus Creator : BusCreator  Inputs=2
  Bus Creator1 : BusCreator  Inputs=6
  Bus Creator{2,4,10..11,16} (5 alike) : BusCreator  Inputs=1
  Bus Creator8 : BusCreator  Inputs=2
  Bus Selector : BusSelector  OutputSignals=Supervisory_Electrical_Out.PON,Supervisory_Electrical_Out.chga_wake,GCM_Electrical_Out.Relay_Charge,GCM_Electrical_Out.Relay_Vehicle
  Constant : Constant
  Constant1 : Constant  Value=0
  Constant10 : Constant  Value=0
  Constant9 : Constant
  EM_Relay : Subsystem
  Engine_Relay : Subsystem
  Ground : Ground
  Relay : Switch  Criteria=u2 > Threshold  Threshold=0.5
  Relay4 : Switch  Criteria=u2 > Threshold  Threshold=0.5
  Terminator : Terminator
  Electrical : Outport
  wires:
  [VNT_Electrical_FromMABx] -> Bus Creator/1
  [VNT_Electrical_FromGCM] -> Bus Creator/2
  Bus Selector/2 -> Bus Creator8/1  "<chga_wake>"
  Relay/1 -> Bus Creator8/2  "BMS_Powerup"
  Bus Creator8/1 -> Bus Creator1/3  "BCM_Electrical"
  Constant9/1 -> Relay4/1
  Bus Selector/4 -> EM_Relay/1(In1), Engine_Relay/1(In1), BAS_Relay/1(In1)  "<Relay_Vehicle>"
  Relay4/1 -> Terminator/1  "Supervisory_Wakeup"
  Constant/1 -> Relay/1
  Constant10/1 -> Relay4/3
  Bus Selector/3 -> Relay/2, Relay4/2  "<Relay_Charge>"
  Constant1/1 -> Relay/3
  Bus Creator/1 -> Bus Selector/1
  Bus Selector/1 -> Bus Creator4/1  "<PON>"
  Bus Creator4/1 -> Bus Creator1/2  "Brusa_Electrical"
  Bus Creator2/1 -> Bus Creator1/1  "Clutch_Trans_Electrical"
  Ground/1 -> Bus Creator2/1  "Dummy1"
  EM_Relay/1(Out1) -> Bus Creator10/1
  Bus Creator10/1 -> Bus Creator1/4  "EM_Electrical"
  Bus Creator11/1 -> Bus Creator1/6  "BAS_Electrical"
  BAS_Relay/1(Out1) -> Bus Creator11/1
  Bus Creator16/1 -> Bus Creator1/5  "ICE_Electrical"
  Engine_Relay/1(Out1) -> Bus Creator16/1
  Bus Creator1/1 -> Electrical/1  "ElectricalRx"

== system EcoSIM3_P2_C2/Powertrain/Soft_ECUs_IO/VNT Vector/ElectricalTx ==
  Electrical : Inport
  Bus Creator : BusCreator  Inputs=7
  Bus Selector1 : BusSelector  OutputSignals=Brusa_Electrical_Out,Clutch_Transmission_Electrical_Out,GM_Electrical_Out,ESS_Electrical_Out,EM_Electrical_Out,BAS_Electrical_Out,ICE_Electrical_Out
  tag scope: VNT_Electrical_From_SoftECU=global
  wires:
  Electrical/1 -> Bus Selector1/1
  Bus Selector1/5 -> Bus Creator/5  "<EM_Electrical_Out>"
  Bus Selector1/6 -> Bus Creator/6  "<BAS_Electrical_Out>"
  Bus Selector1/3 -> Bus Creator/3  "<GM_Electrical_Out>"
  Bus Selector1/7 -> Bus Creator/7  "<ICE_Electrical_Out>"
  Bus Selector1/4 -> Bus Creator/4  "<ESS_Electrical_Out>"
  Bus Selector1/1 -> Bus Creator/1  "<Brusa_Electrical_Out>"
  Bus Selector1/2 -> Bus Creator/2  "<Clutch_Transmission_Electrical_Out>"
  Bus Creator/1 -> [VNT_Electrical_From_SoftECU]  "From_SoftECU"

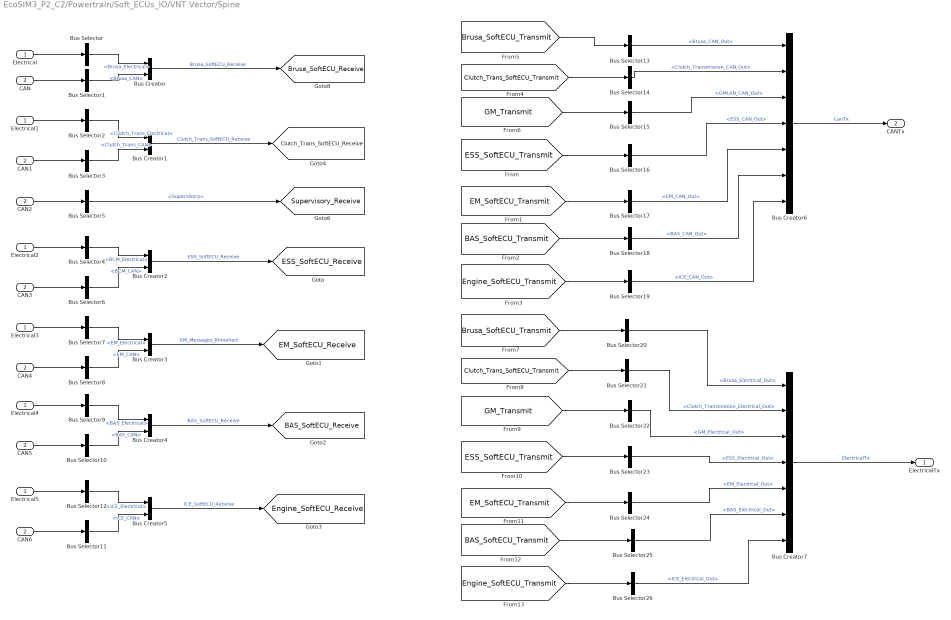
== system EcoSIM3_P2_C2/Powertrain/Soft_ECUs_IO/VNT Vector/Spine ==
  Electrical : Inport
  CAN : Inport  Port=2
  Bus Creator{,1..5} (6 alike) : BusCreator  Inputs=2
  Bus Creator6 : BusCreator  Inputs=7
  Bus Creator7 : BusCreator  Inputs=7
  Bus Selector : BusSelector  OutputSignals=Brusa_Electrical
  Bus Selector1 : BusSelector  OutputSignals=Brusa_CAN
  Bus Selector10 : BusSelector  OutputSignals=BAS_CAN
  Bus Selector11 : BusSelector  OutputSignals=ICE_CAN
  Bus Selector12 : BusSelector  OutputSignals=ICE_Electrical
  Bus Selector13 : BusSelector  OutputSignals=Brusa_CAN_Out
  Bus Selector14 : BusSelector  OutputSignals=Clutch_Transmission_CAN_Out
  Bus Selector15 : BusSelector  OutputSignals=GMLAN_CAN_Out
  Bus Selector16 : BusSelector  OutputSignals=ESS_CAN_Out
  Bus Selector17 : BusSelector  OutputSignals=EM_CAN_Out
  Bus Selector18 : BusSelector  OutputSignals=BAS_CAN_Out
  Bus Selector19 : BusSelector  OutputSignals=ICE_CAN_Out
  Bus Selector2 : BusSelector  OutputSignals=Clutch_Trans_Electrical
  Bus Selector20 : BusSelector  OutputSignals=Brusa_Electrical_Out
  Bus Selector21 : BusSelector  OutputSignals=Clutch_Transmission_Electrical_Out
  Bus Selector22 : BusSelector  OutputSignals=GM_Electrical_Out
  Bus Selector23 : BusSelector  OutputSignals=ESS_Electrical_Out
  Bus Selector24 : BusSelector  OutputSignals=EM_Electrical_Out
  Bus Selector25 : BusSelector  OutputSignals=BAS_Electrical_Out
  Bus Selector26 : BusSelector  OutputSignals=ICE_Electrical_Out
  Bus Selector3 : BusSelector  OutputSignals=Clutch_Trans_CAN
  Bus Selector4 : BusSelector  OutputSignals=BCM_Electrical
  Bus Selector5 : BusSelector  OutputSignals=Supervisory
  Bus Selector6 : BusSelector  OutputSignals=BCM_CAN
  Bus Selector7 : BusSelector  OutputSignals=EM_Electrical
  Bus Selector8 : BusSelector  OutputSignals=EM_CAN
  Bus Selector9 : BusSelector  OutputSignals=BAS_Electrical
  CAN{1..6} (6 alike) : InportShadow  Port=2
  Electrical{1..5} (5 alike) : InportShadow
  ElectricalTx : Outport
  CANTx : Outport  Port=2
  tag scope: BAS_SoftECU_Receive=global, Brusa_SoftECU_Receive=global, Clutch_Trans_SoftECU_Receive=global, EM_SoftECU_Receive=global, ESS_SoftECU_Receive=global, Engine_SoftECU_Receive=global, Supervisory_Receive=global
  wires:
  Electrical/1 -> Bus Selector/1
  CAN/1 -> Bus Selector1/1
  Bus Selector/1 -> Bus Creator/1  "<Brusa_Electrical>"
  Bus Selector1/1 -> Bus Creator/2  "<Brusa_CAN>"
  Bus Creator/1 -> [Brusa_SoftECU_Receive]  "Brusa_SoftECU_Receive"
  Electrical1/1 -> Bus Selector2/1
  CAN1/1 -> Bus Selector3/1
  Bus Selector2/1 -> Bus Creator1/1  "<Clutch_Trans_Electrical>"
  Bus Selector3/1 -> Bus Creator1/2  "<Clutch_Trans_CAN>"
  Bus Creator1/1 -> [Clutch_Trans_SoftECU_Receive]  "Clutch_Trans_SoftECU_Receive"
  CAN2/1 -> Bus Selector5/1
  Bus Selector5/1 -> [Supervisory_Receive]  "<Supervisory>"
  Electrical2/1 -> Bus Selector4/1
  CAN3/1 -> Bus Selector6/1
  Bus Selector4/1 -> Bus Creator2/1  "<BCM_Electrical>"
  Bus Selector6/1 -> Bus Creator2/2  "<BCM_CAN>"
  Bus Creator2/1 -> [ESS_SoftECU_Receive]  "ESS_SoftECU_Receive"
  Electrical3/1 -> Bus Selector7/1
  CAN4/1 -> Bus Selector8/1
  Bus Selector7/1 -> Bus Creator3/1  "<EM_Electrical>"
  Bus Selector8/1 -> Bus Creator3/2  "<EM_CAN>"
  Bus Creator3/1 -> [EM_SoftECU_Receive]  "EM_Messages_Rhinehart"
  Electrical4/1 -> Bus Selector9/1
  CAN5/1 -> Bus Selector10/1
  Bus Selector9/1 -> Bus Creator4/1  "<BAS_Electrical>"
  Bus Selector10/1 -> Bus Creator4/2  "<BAS_CAN>"
  Bus Creator4/1 -> [BAS_SoftECU_Receive]  "BAS_SoftECU_Receive"
  Electrical5/1 -> Bus Selector12/1
  CAN6/1 -> Bus Selector11/1
  Bus Selector12/1 -> Bus Creator5/1  "<ICE_Electrical>"
  Bus Selector11/1 -> Bus Creator5/2  "<ICE_CAN>"
  Bus Creator5/1 -> [Engine_SoftECU_Receive]  "ICE_SoftECU_Receive"
  [Brusa_SoftECU_Transmit] -> Bus Selector13/1
  [Clutch_Trans_SoftECU_Transmit] -> Bus Selector14/1
  [GM_Transmit] -> Bus Selector15/1
  [ESS_SoftECU_Transmit] -> Bus Selector16/1
  [EM_SoftECU_Transmit] -> Bus Selector17/1
  [BAS_SoftECU_Transmit] -> Bus Selector18/1
  [Engine_SoftECU_Transmit] -> Bus Selector19/1
  Bus Selector13/1 -> Bus Creator6/1  "<Brusa_CAN_Out>"
  Bus Selector14/1 -> Bus Creator6/2  "<Clutch_Transmission_CAN_Out>"
  Bus Selector15/1 -> Bus Creator6/3  "<GMLAN_CAN_Out>"
  Bus Selector16/1 -> Bus Creator6/4  "<ESS_CAN_Out>"
  Bus Selector17/1 -> Bus Creator6/5  "<EM_CAN_Out>"
  Bus Selector18/1 -> Bus Creator6/6  "<BAS_CAN_Out>"
  Bus Selector19/1 -> Bus Creator6/7  "<ICE_CAN_Out>"
  [Brusa_SoftECU_Transmit] -> Bus Selector20/1
  [Clutch_Trans_SoftECU_Transmit] -> Bus Selector21/1
  [GM_Transmit] -> Bus Selector22/1
  [ESS_SoftECU_Transmit] -> Bus Selector23/1
  [EM_SoftECU_Transmit] -> Bus Selector24/1
  [BAS_SoftECU_Transmit] -> Bus Selector25/1
  [Engine_SoftECU_Transmit] -> Bus Selector26/1
  Bus Selector20/1 -> Bus Creator7/1  "<Brusa_Electrical_Out>"
  Bus Selector21/1 -> Bus Creator7/2  "<Clutch_Transmission_Electrical_Out>"
  Bus Selector22/1 -> Bus Creator7/3  "<GM_Electrical_Out>"
  Bus Selector23/1 -> Bus Creator7/4  "<ESS_Electrical_Out>"
  Bus Selector24/1 -> Bus Creator7/5  "<EM_Electrical_Out>"
  Bus Selector25/1 -> Bus Creator7/6  "<BAS_Electrical_Out>"
  Bus Selector26/1 -> Bus Creator7/7  "<ICE_Electrical_Out>"
  Bus Creator7/1 -> ElectricalTx/1  "ElectricalTx"
  Bus Creator6/1 -> CANTx/1  "CanTx"

== system EcoSIM3_P2_C2/Powertrain/Vehicle Dynamics/Sensor/Sensor lag ==
  i : Inport
  1st Order LPF of 1ms in Discrete Form : DiscreteTransferFcn  Numerator=[0.6321]  Denominator=[1 -0.3679]
  o : Outport
  wires:
  i/1 -> 1st Order LPF of 1ms in Discrete Form/1
  1st Order LPF of 1ms in Discrete Form/1 -> o/1

== system EcoSIM3_P2_C2/Powertrain/Vehicle Dynamics/Sensor/Sensor lag1 ==
  i : Inport
  1st Order LPF of 1ms in Discrete Form : DiscreteTransferFcn  Numerator=[0.6321]  Denominator=[1 -0.3679]
  o : Outport
  wires:
  1st Order LPF of 1ms in Discrete Form/1 -> o/1
  i/1 -> 1st Order LPF of 1ms in Discrete Form/1

== system EcoSIM3_P2_C2/Powertrain/Vehicle Dynamics/Sensor/Sensor lag2 ==
  i : Inport
  1st Order LPF of 1ms in Discrete Form : DiscreteTransferFcn  Numerator=[0.6321]  Denominator=[1 -0.3679]
  o : Outport
  wires:
  i/1 -> 1st Order LPF of 1ms in Discrete Form/1
  1st Order LPF of 1ms in Discrete Form/1 -> o/1

== system EcoSIM3_P2_C2/Powertrain/Vehicle Dynamics/Sensor/Sensor lag3 ==
  i : Inport
  1st Order LPF of 1ms in Discrete Form : DiscreteTransferFcn  Numerator=[0.6321]  Denominator=[1 -0.3679]
  o : Outport
  wires:
  i/1 -> 1st Order LPF of 1ms in Discrete Form/1
  1st Order LPF of 1ms in Discrete Form/1 -> o/1

== system EcoSIM3_P2_C2/Powertrain/Vehicle Dynamics/Sensor/Sensor lag4 ==
  i : Inport
  1st Order LPF of 1ms in Discrete Form : DiscreteTransferFcn  Numerator=[0.6321]  Denominator=[1 -0.3679]
  o : Outport
  wires:
  1st Order LPF of 1ms in Discrete Form/1 -> o/1
  i/1 -> 1st Order LPF of 1ms in Discrete Form/1

== system EcoSIM3_P2_C2/RTI Data/RTI Data Store/RTI Data Store/RTI Data Store ==
  RTI Data Store : Subsystem  mask(RTI_DATA_STORE){}
      mask help:
      | RTI Data Store Block. This block is used by RTI to store internal model dependent data. Deleting this block will result in data loss.
      |
      | NEVER DELETE, COPY, OR MODIFY THIS BLOCK!
      mask Help:
      | RTI Data Store Block. This block is used by RTI to store internal model dependent data. Deleting this block will result in data loss.
      | 
      | NEVER DELETE, COPY, OR MODIFY THIS BLOCK!
      mask Display: text(0.5, 0.5, ' ', 'HorizontalAlignment', 'center');

== system EcoSIM3_P2_C2/Supervisory Controller/Functional Safety1/Functional Safety Algorithm/Fault Detection (Team Developed) ==
  Torque Requests : Inport
  ECU/Sensor Signals : Inport  Port=2
  Accelerator Pedal Faults : Subsystem  Commented=on
  Brake Pedal Faults : Subsystem  Commented=on
  Bus Creator : BusCreator  Inputs=5
  Drivetrain Faults : Subsystem  Commented=on
  Parking Brake Faults : Subsystem  Commented=on
  Torque Security Faults : Subsystem
  Team Dev Fault Signals : Outport
  wires:
  Torque Security Faults/1(Faults) -> Bus Creator/1
  Accelerator Pedal Faults/1(Out1) -> Bus Creator/2
  Brake Pedal Faults/1(Out1) -> Bus Creator/3
  Torque Requests/1 -> Torque Security Faults/1(Torque Requests)
  Drivetrain Faults/1(Out1) -> Bus Creator/5
  Parking Brake Faults/1(Out1) -> Bus Creator/4
  ECU/Sensor Signals/1 -> Torque Security Faults/2(ECU/Sensor Signals), Accelerator Pedal Faults/1(In1), Brake Pedal Faults/1(In1), Parking Brake Faults/1(In1), Drivetrain Faults/1(In1)
  Bus Creator/1 -> Team Dev Fault Signals/1  "Team_Dev_Faults"

== system EcoSIM3_P2_C2/Supervisory Controller/Functional Safety1/Functional Safety Algorithm/Fault Management ==
  Team Dev Fault Signals : Inport
  ECU/Sensor Signals : Inport  Port=2
  Bus Selector : BusSelector  OutputSignals=Trq_Security_Faults.EM_Trq_Fault
  Data Type Conversion : DataTypeConversion
  Gain : Gain
  Terminator : Terminator
  Truth Table : Truth Table  Commented=on  TreatAsAtomicUnit=on
  Fault Code : Outport
  wires:
  Bus Selector/1 -> Gain/1  "<EM_Trq_Fault>"
  ECU/Sensor Signals/1 -> Terminator/1
  Team Dev Fault Signals/1 -> Bus Selector/1
  Data Type Conversion/1 -> Fault Code/1  "hsc_FS_Fault_Code"
  Gain/1 -> Data Type Conversion/1  "hsc_FS_Fault_Code"

== system EcoSIM3_P2_C2/Supervisory Controller/Functional Safety1/Functional Safety Algorithm/Fault Mitigation ==
  Fault Code : Inport
  1-D Lookup Table : Lookup_n-D  NumberOfTableDimensions=1  BreakpointsForDimension1=[0 1]  Table=[1 1]  InterpMethod=Nearest  InternalRulePriority=Speed  RndMeth=Simplest  InputSameDT=on
  1-D Lookup Table1 : Lookup_n-D  NumberOfTableDimensions=1  BreakpointsForDimension1=[0 1]  Table=[1 1]  InterpMethod=Nearest  InternalRulePriority=Speed  RndMeth=Simplest  InputSameDT=on
  1-D Lookup Table2 : Lookup_n-D  NumberOfTableDimensions=1  BreakpointsForDimension1=[0 1]  Table=[1 0]  InterpMethod=Nearest  InternalRulePriority=Speed  RndMeth=Simplest  InputSameDT=on
  Bus Creator : BusCreator  Inputs=3
  Torque Limits : Outport
  wires:
  1-D Lookup Table2/1 -> Bus Creator/3  "EM_Trq_Limit"
  1-D Lookup Table1/1 -> Bus Creator/2  "Eng_Trq_Limit"
  1-D Lookup Table/1 -> Bus Creator/1  "BAS_Trq_Limit"
  Bus Creator/1 -> Torque Limits/1  "Fault_Torque_Limits"
  Fault Code/1 -> 1-D Lookup Table/1, 1-D Lookup Table1/1, 1-D Lookup Table2/1

== system EcoSIM3_P2_C2/Supervisory Controller/Input Conditioning/Velocity Conditioning/Subsystem ==
  In1 : Inport
  Add : Sum  Inputs=+-
  Delay : Delay  DelayLength=50
  Derivative : Derivative
  Gain6 : Gain  Gain=2*pi
  Memory : Memory
  Memory2 : Memory
  Product : Product
  Product1 : Product  Inputs=*/
  Product2 : Product  Inputs=*/
  Product3 : Product  Inputs=*/
  Product4 : Product
  Saturation : Saturate  UpperLimit=inf  LowerLimit=0
  Scope8 : Scope
      settings: SaveName=ScopeData21
  Switch : Switch
  Switch2 : Switch
  Terminator : Terminator
  Ticks_per_rev : Constant  Value=48
  TimeDiff : Constant  Value=0.5
  Transfer Fcn : TransferFcn  Numerator=[4]  Denominator=[1 4]
  Transfer Fcn1 : TransferFcn  Numerator=[4]  Denominator=[1 4]
  Tyre_rad_m : Constant  Value=Plants.Rear_wh.Tire.rollrad
  m/s to km/hr : Gain  Gain=1/1000*3600
  m/s to km/hr1 : Gain  Gain=1/1000*3600
  Speed_LD : Outport
  wires:
  Switch/1 -> Transfer Fcn/1, Memory/1
  Derivative/1 -> Switch/1, Switch/2
  Memory/1 -> Switch/3
  Transfer Fcn/1 -> Saturation/1
  Saturation/1 -> Product1/1
  Product1/1 -> Product/1
  Product/1 -> m/s to km/hr/1  "Left_Driven_m_per_sec"
  m/s to km/hr/1 -> Terminator/1
  Ticks_per_rev/1 -> Product3/2, Product1/2
  Tyre_rad_m/1 -> Gain6/1
  In1/1 -> Derivative/1, Add/1, Delay/1
  Switch2/1 -> Transfer Fcn1/1, Memory2/1
  Product4/1 -> Speed_LD/1, m/s to km/hr1/1  "Left_Driven_mps_delay"
  Delay/1 -> Add/2
  Product2/1 -> Switch2/2, Switch2/1
  TimeDiff/1 -> Product2/2
  Memory2/1 -> Switch2/3
  Transfer Fcn1/1 -> Product3/1
  m/s to km/hr1/1 -> Scope8/1  "Left_Driven_kph"
  Gain6/1 -> Product4/2, Product/2
  Product3/1 -> Product4/1
  Add/1 -> Product2/1

== system EcoSIM3_P2_C2/Supervisory Controller/Input Conditioning/Velocity Conditioning/Subsystem1 ==
  In1 : Inport
  Add : Sum  Inputs=+-
  Delay : Delay  DelayLength=50
  Gain6 : Gain  Gain=2*pi
  Memory2 : Memory
  Product2 : Product  Inputs=*/
  Product3 : Product  Inputs=*/
  Product4 : Product
  Scope8 : Scope
      settings: SaveName=ScopeData21
  Switch2 : Switch
  Ticks_per_rev : Constant  Value=48
  TimeDiff : Constant  Value=0.5
  Transfer Fcn1 : TransferFcn  Numerator=[4]  Denominator=[1 4]
  Tyre_rad_m : Constant  Value=Plants.Rear_wh.Tire.rollrad
  m/s to km/hr1 : Gain  Gain=1/1000*3600
  Speed_RD : Outport
  wires:
  Add/1 -> Product2/1
  Product3/1 -> Product4/1
  Gain6/1 -> Product4/2
  m/s to km/hr1/1 -> Scope8/1  "Right_Driven_kph"
  Transfer Fcn1/1 -> Product3/1
  Memory2/1 -> Switch2/3
  TimeDiff/1 -> Product2/2
  Product2/1 -> Switch2/1, Switch2/2
  Delay/1 -> Add/2
  Product4/1 -> m/s to km/hr1/1, Speed_RD/1  "Right_Driven_mps_delay"
  Switch2/1 -> Memory2/1, Transfer Fcn1/1
  In1/1 -> Delay/1, Add/1
  Tyre_rad_m/1 -> Gain6/1
  Ticks_per_rev/1 -> Product3/2

== system EcoSIM3_P2_C2/Supervisory Controller/Input Conditioning/Velocity Conditioning/Subsystem2 ==
  In1 : Inport
  Add : Sum  Inputs=+-
  Delay : Delay  DelayLength=50
  Gain6 : Gain  Gain=2*pi
  Memory2 : Memory
  Product2 : Product  Inputs=*/
  Product3 : Product  Inputs=*/
  Product4 : Product
  Scope8 : Scope
      settings: SaveName=ScopeData21
  Switch2 : Switch
  Ticks_per_rev : Constant  Value=48
  TimeDiff : Constant  Value=0.5
  Transfer Fcn1 : TransferFcn  Numerator=[4]  Denominator=[1 4]
  Tyre_rad_m : Constant  Value=Plants.Rear_wh.Tire.rollrad
  m/s to km/hr1 : Gain  Gain=1/1000*3600
  Speed_LND : Outport
  wires:
  Ticks_per_rev/1 -> Product3/2
  Tyre_rad_m/1 -> Gain6/1
  In1/1 -> Add/1, Delay/1
  Switch2/1 -> Transfer Fcn1/1, Memory2/1
  Product4/1 -> Speed_LND/1, m/s to km/hr1/1  "Left_NonDriven_mps_delay"
  Delay/1 -> Add/2
  Product2/1 -> Switch2/2, Switch2/1
  TimeDiff/1 -> Product2/2
  Memory2/1 -> Switch2/3
  Transfer Fcn1/1 -> Product3/1
  m/s to km/hr1/1 -> Scope8/1  "Left_NonDriven_kph"
  Gain6/1 -> Product4/2
  Product3/1 -> Product4/1
  Add/1 -> Product2/1

== system EcoSIM3_P2_C2/Supervisory Controller/Input Conditioning/Velocity Conditioning/Subsystem3 ==
  In1 : Inport
  Add : Sum  Inputs=+-
  Delay : Delay  DelayLength=50
  Gain6 : Gain  Gain=2*pi
  Memory2 : Memory
  Product2 : Product  Inputs=*/
  Product3 : Product  Inputs=*/
  Product4 : Product
  Scope8 : Scope
      settings: SaveName=ScopeData21
  Switch2 : Switch
  Ticks_per_rev : Constant  Value=48
  TimeDiff : Constant  Value=0.5
  Transfer Fcn1 : TransferFcn  Numerator=[4]  Denominator=[1 4]
  Tyre_rad_m : Constant  Value=Plants.Rear_wh.Tire.rollrad
  m/s to km/hr1 : Gain  Gain=1/1000*3600
  Speed_RND : Outport
  wires:
  Add/1 -> Product2/1
  Product3/1 -> Product4/1
  Gain6/1 -> Product4/2
  m/s to km/hr1/1 -> Scope8/1  "Right_NonDriven_kph"
  Transfer Fcn1/1 -> Product3/1
  Memory2/1 -> Switch2/3
  TimeDiff/1 -> Product2/2
  Product2/1 -> Switch2/1, Switch2/2
  Delay/1 -> Add/2
  Product4/1 -> m/s to km/hr1/1, Speed_RND/1  "Right_NonDriven_mps_delay"
  Switch2/1 -> Memory2/1, Transfer Fcn1/1
  In1/1 -> Delay/1, Add/1
  Tyre_rad_m/1 -> Gain6/1
  Ticks_per_rev/1 -> Product3/2

== system EcoSIM3_P2_C2/Supervisory Controller/Mode Operation/Accessory/BAS_Signals ==
  Bus Creator4 : BusCreator  Inputs=3
  Constant1 : Constant  Value=0
  Constant4 : Constant  Value=0
  Constant5 : Constant  Value=0
  Out1 : Outport
  wires:
  Constant5/1 -> Bus Creator4/3  "BAS_Mode_Request"
  Constant4/1 -> Bus Creator4/1  "BAS_Torque_Request_Nm"
  Bus Creator4/1 -> Out1/1  "BAS_SoftECU_Receive"
  Constant1/1 -> Bus Creator4/2  "BAS_Speed_Request"

== system EcoSIM3_P2_C2/Supervisory Controller/Mode Operation/Accessory/DC//DC Enabled ==
  Bus Creator : BusCreator  Inputs=3
  Constant : Constant
  Constant1 : Constant  Value=12.8
  Constant2 : Constant
  Out1 : Outport
  wires:
  Constant/1 -> Bus Creator/1  "LowVoltEnablRq"
  Constant1/1 -> Bus Creator/2  "LwVltStpntCmnd"
  Constant2/1 -> Bus Creator/3  "PrplsnSysAtv"
  Bus Creator/1 -> Out1/1  "DC_DC"
